simulink subsystem "DMPC"  (R2023a)
settings: Solver=VariableStepAuto  StartTime=0.0  StopTime=10.0  RelTol=1e-3
settings Model: Creator=giaco  LastModifiedBy=giaco

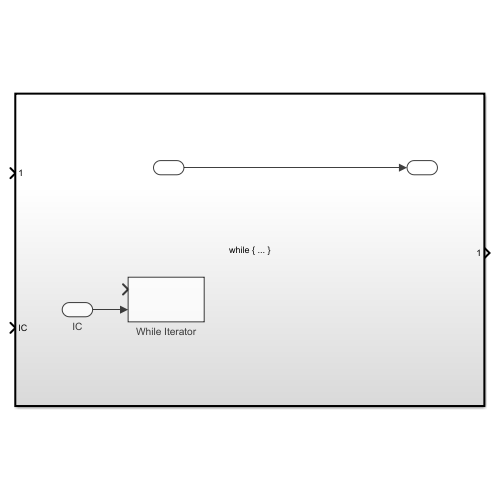
[thumbnail: Simulink's stored preview of the top-level diagram]
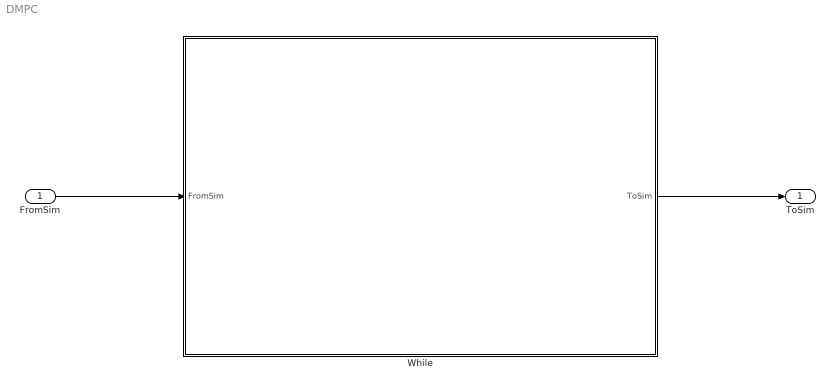
== system DMPC ==
  FromSim : Inport
  While : Subsystem  TreatAsAtomicUnit=on
  ToSim : Outport
  wires:
  FromSim/1 -> While/1(FromSim)
  While/1(ToSim) -> ToSim/1

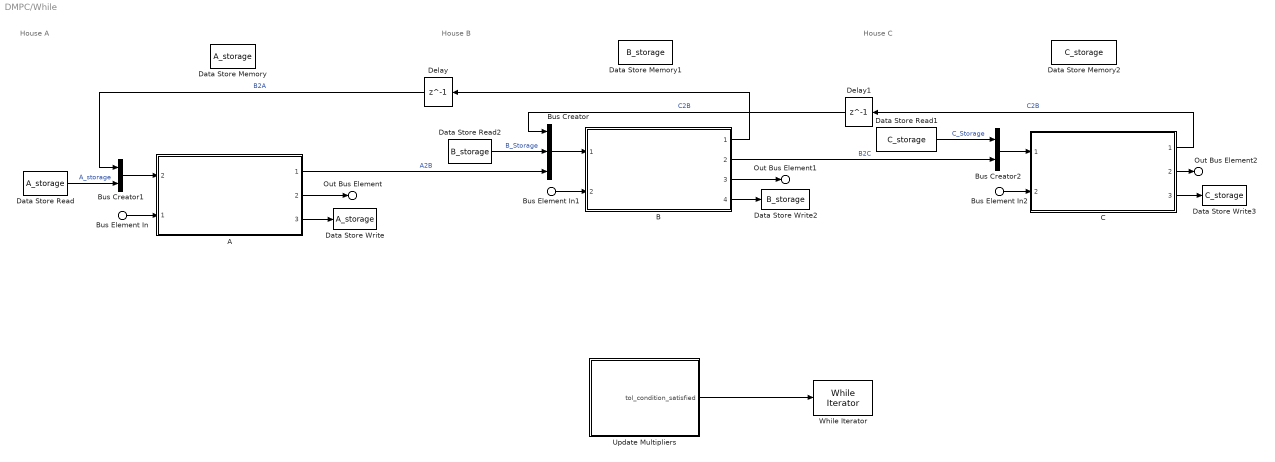
== system DMPC/While ==
  note: House C
  note: House A
  note: House B
  Bus Element In : Inport  PortName=FromSim  Element=HouseA
  Bus Element In1 : Inport  PortName=FromSim  Element=HouseB
  Bus Element In2 : Inport  PortName=FromSim  Element=HouseC
  A : Subsystem  ReferencedSubsystem=FirstHouse
      settings: PortSchema="{\"entries\":[{\"content\":{\"sides\":[{\"content\":{\"connectorIds\":[\"In2\",\"In1\"]},\"type\":\"ConnectorPlacement.EquallySpacedRectSide\",\"uuid\":\"84563440-d2af-48f4-950c-3cdf3e12c99b\"},{\"content\":{\"connectorIds\":[\"Out1\",\"Out2\",\"Out3\"],\"side\":\"RIGHT\"},\"type\":\"ConnectorPlacement.EquallySpacedRectSide\",\"uuid\":\"a87ee087-c02f-49a0-bc4b-c3a416de0173\"},{\"content\":{\"side\":\"TOP\"},\"type\":\"ConnectorPlacement.EquallySpacedRectSide\",\"uuid\":\"e4de9a36-35d0-4055-a23e-40ce8dd64b27\"}]},\"type\":\"ConnectorPlacement.EquallySpacedConnector\",\"uuid\":\"d0abf100-c86f-42b9-be19-ed721fbf1cc7\"}],\"packageUris\":[\"http://schema.mathworks.com/mf0/Connector/R2020b\"],\"version\":\"1.0\"}"
  B : Subsystem  ReferencedSubsystem=MiddleHouse
  Bus Creator : BusCreator  Inputs=3
  Bus Creator1 : BusCreator  Inputs=2
  Bus Creator2 : BusCreator  Inputs=2
  C : Subsystem  ReferencedSubsystem=BypassHouse
  Data Store Memory : DataStoreMemory  DataStoreName=A_storage  WriteAfterWriteMsg=warning  ShowAdditionalParam=off  OutDataTypeStr=Bus: NMPC_A_output
  Data Store Memory1 : DataStoreMemory  DataStoreName=B_storage  WriteAfterWriteMsg=warning  ShowAdditionalParam=off  OutDataTypeStr=Bus: NMPC_B_output
  Data Store Memory2 : DataStoreMemory  DataStoreName=C_storage  WriteAfterWriteMsg=warning  ShowAdditionalParam=off  OutDataTypeStr=Bus: NMPC_C_output
  Data Store Read : DataStoreRead  DataStoreName=A_storage  IndexOptions=Index vector (dialog)  Indices=1  OutputSizes=1
  Data Store Read1 : DataStoreRead  DataStoreName=C_storage  IndexOptions=Index vector (dialog)  Indices=1  OutputSizes=1
  Data Store Read2 : DataStoreRead  DataStoreName=B_storage  IndexOptions=Index vector (dialog)  Indices=1  OutputSizes=1
  Data Store Write : DataStoreWrite  DataStoreName=A_storage  IndexOptions=Index vector (dialog)  Indices=1  OutputSizes=1
  Data Store Write2 : DataStoreWrite  DataStoreName=B_storage  IndexOptions=Index vector (dialog)  Indices=1  OutputSizes=1
  Data Store Write3 : DataStoreWrite  DataStoreName=C_storage  IndexOptions=Index vector (dialog)  Indices=1  OutputSizes=1
  Delay : Delay  DelayLength=1
  Delay1 : Delay  DelayLength=1
  Update Multipliers : MATLAB Function  TreatAsAtomicUnit=on
  While Iterator : WhileIterator  MaxIters=1000  WhileBlockType=do-while
  Out Bus Element : Outport  PortName=ToSim  Element=HouseA
  Out Bus Element1 : Outport  PortName=ToSim  Element=HouseB
  Out Bus Element2 : Outport  PortName=ToSim  Element=HouseC
  wires:
  Bus Creator1/1 -> A/2
  Delay1/1 -> Bus Creator/1  "C2B"
  Delay/1 -> Bus Creator1/1  "B2A"
  Bus Creator2/1 -> C/1
  Data Store Read1/1 -> Bus Creator2/1  "C_Storage"
  C/2 -> Out Bus Element2/1
  Bus Element In/1 -> A/1
  C/3 -> Data Store Write3/1
  B/4 -> Data Store Write2/1
  Data Store Read2/1 -> Bus Creator/2  "B_Storage"
  Data Store Read/1 -> Bus Creator1/2  "A_storage"
  A/3 -> Data Store Write/1
  B/1 -> Delay/1
  B/3 -> Out Bus Element1/1
  C/1 -> Delay1/1  "C2B"
  B/2 -> Bus Creator2/2  "B2C"
  Bus Creator/1 -> B/1
  A/1 -> Bus Creator/3  "A2B"
  A/2 -> Out Bus Element/1
  Update Multipliers/1(tol_condition_satisfied) -> While Iterator/1
  Bus Element In2/1 -> C/2
  Bus Element In1/1 -> B/2

== matlab function DMPC/While/Update Multipliers ==
  data: tol_condition_satisfied output boolean; A_storage data_store_memory; B_storage data_store_memory; C_storage data_store_memory
function tol_condition_satisfied  = fcn

global A_storage
global B_storage
global C_storage

persistent difference
if isempty(difference)
    difference = struct();
end

%%
tol_condition = 1;

%% A-B Lagrange Multiplier Update  

% lambda_AB_m_O
A_storage.md_seq.lambda_m_O_B_A = A_storage.md_seq.lambda_m_O_B_A + A.alfa_m_O_succ * (A_storage.mv_seq.m_O_A_A - A_storage.md_seq.m_O_A_B);
B_storage.md_seq.lambda_m_O_A_B = B_storage.md_seq.lambda_m_O_A_B + B.alfa_m_O_pred * (B_storage.md_seq.m_O_A_A - B_storage.mv_seq.m_F_B_B);
% lambda_storage.lambda_AB_m_O = lambda_storage.lambda_AB_m_O + A/B/..alfa.m_O * (A_storage.mv_seq.m_O_A_A - A_storage.mv_seq.m_O_B_B)

if any(A_storage.md_seq.lambda_m_O_B_A ~= B_storage.md_seq.lambda_m_O_A_B)
    error('The updated lambdas are not equal.');
end

difference.m_O_AB = norm((A_storage.mv_seq.m_O_A_A - A_storage.md_seq.m_O_A_B));

% lambda_AB_T_F
A_storage.md_seq.lambda_T_F_B_A = A_storage.md_seq.lambda_T_F_B_A + A.alfa_T_F_succ * (A_storage.mv_seq.T_F_A_A - A_storage.md_seq.T_F_A_B);
B_storage.md_seq.lambda_T_F_A_B = B_storage.md_seq.lambda_T_F_A_B + B.alfa_T_F_pred * (B_storage.md_seq.T_F_A_A - B_storage.mv_seq.T_F_A_B);

if any(A_storage.md_seq.lambda_T_F_B_A ~= B_storage.md_seq.lambda_T_F_A_B)
    error('The updated lambdas are not equal.');
end

difference.T_F_AB = norm((A_storage.mv_seq.T_F_A_A - A_storage.md_seq.T_F_A_B));

% lambda_AB_m_R
A_storage.md_seq.lambda_m_R_B_A = A_storage.md_seq.lambda_m_R_B_A + A.alfa_m_R_succ * (A_storage.mv_seq.m_R_B_A - A_storage.md_seq.m_R_B_B);
B_storage.md_seq.lambda_m_R_A_B = B_storage.md_seq.lambda_m_R_A_B + B.alfa_m_R_pred * (B_storage.md_seq.m_R_B_A - B_storage.mv_seq.m_R_B_B);

if any(A_storage.md_seq.lambda_m_R_B_A  ~= B_storage.md_seq.lambda_m_R_A_B)
    error('The updated lambdas are not equal.');
end

difference.m_R_AB = norm((A_storage.mv_seq.m_R_B_A - A_storage.md_seq.m_R_B_B));

% lambda_AB_T_R
A_storage.md_seq.lambda_T_R_B_A = A_storage.md_seq.lambda_T_R_B_A + A.alfa_T_R_succ * (A_storage.mv_seq.T_R_B_A - A_storage.md_seq.T_R_B_B);
B_storage.md_seq.lambda_T_R_A_B = B_storage.md_seq.lambda_T_R_A_B + B.alfa_T_R_pred * (B_storage.md_seq.T_R_B_A - B_storage.mv_seq.T_R_B_B);

if any(A_storage.md_seq.lambda_T_R_B_A  ~= B_storage.md_seq.lambda_T_R_A_B)
    error('The updated lambdas are not equal.');
end

difference.T_R_AB = norm((A_storage.mv_seq.T_R_B_A - A_storage.md_seq.T_R_B_B));

%% B-C Lagrange Multiplier Update

% lambda_BC_m_O
B_storage.md_seq.lambda_m_O_C_B = A_storage.md_seq.lambda_m_O_C_B + B.alfa_m_O_succ * (B_storage.mv_seq.m_O_B_B - B_storage.md_seq.m_O_B_C);
C_storage.md_seq.lambda_m_O_B_C = B_storage.md_seq.lambda_m_O_B_C + C.alfa_m_O_pred * (C_storage.md_seq.m_O_B_B - C_storage.mv_seq.m_F_C_C);
% lambda_storage.lambda_AB_m_O = lambda_storage.lambda_AB_m_O + A/B/..alfa.m_O * (A_storage.mv_seq.m_O_A_A - A_storage.mv_seq.m_O_B_B)

if any(B_storage.md_seq.lambda_m_O_C_B  ~= C_storage.md_seq.lambda_m_O_B_C)
    error('The updated lambdas are not equal.');
end

difference.m_F_BC = norm((B_storage.mv_seq.m_O_B_B - B_storage.md_seq.m_O_B_C));

% lambda_CB_T_F
B_storage.md_seq.lambda_T_F_C_B = B_storage.md_seq.lambda_T_F_C_B + B.alfa_T_F_succ * (B_storage.mv_seq.T_F_B_B - B_storage.md_seq.T_F_B_C);
C_storage.md_seq.lambda_T_F_B_C = C_storage.md_seq.lambda_T_F_B_C + C.alfa_T_F_pred * (C_storage.md_seq.T_F_B_B - C_storage.mv_seq.T_F_B_C);

if any(B_storage.md_seq.lambda_T_F_C_B  ~= C_storage.md_seq.lambda_T_F_B_C)
    error('The updated lambdas are not equal.');
end

difference.T_F_BC = norm((B_storage.mv_seq.T_F_B_B - B_storage.md_seq.T_F_B_C));

% lambda_CB_m_R
B_storage.md_seq.lambda_m_R_C_B = B_storage.md_seq.lambda_m_R_C_B + B.alfa_m_R_succ * (B_storage.mv_seq.m_R_C_B - B_storage.md_seq.m_R_C_C);
C_storage.md_seq.lambda_m_R_B_C = C_storage.md_seq.lambda_m_R_B_C + C.alfa_m_R_pred * (C_storage.md_seq.m_R_C_B - C_storage.mv_seq.m_R_C_C);

if any(B_storage.md_seq.lambda_m_R_C_B  ~= C_storage.md_seq.lambda_m_R_B_C)
    error('The updated lambdas are not equal.');
end

difference.m_R_BC = norm((B_storage.mv_seq.m_R_C_B - B_storage.md_seq.m_R_C_C));

% lambda_CB_T_R
B_storage.md_seq.lambda_T_R_C_B = B_storage.md_seq.lambda_T_R_C_B + B.alfa_T_R_succ * (B_storage.mv_seq.T_R_C_B - B_storage.md_seq.T_R_C_C);
C_storage.md_seq.lambda_T_R_B_C = C_storage.md_seq.lambda_T_R_B_C + C.alfa_T_R_pred * (C_storage.md_seq.T_R_C_B - C_storage.mv_seq.T_R_C_C);

if any(B_storage.md_seq.lambda_T_R_C_B  ~= C_storage.md_seq.lambda_T_R_B_C)
    error('The updated lambdas are not equal.');
end

difference.m_R_BC = norm((B_storage.mv_seq.T_R_C_B - B_storage.md_seq.T_R_C_C));

%% Condition check 

norm_sum = 0;
fields = fieldnames(difference);
for i = 1:numel(fields)
    norm_sum = norm_sum + difference.(fields{i});
end

if norm_sum <= tol_condition
    tol_condition_satisfied = true;
else
    tol_condition_satisfied = false;
end
